simulink model "DTNS_KAISIM_V2"  (R2022a)
settings: Solver=FixedStepDiscrete  StartTime=0.0  StopTime=500  FixedStep=0.04  RelTol=1e-3
PreLoadFcn:
  | listing = dir;
  | if (contains([listing .name], 'DTNS_KAISIM_V2.slx'))
  |     addpath('./TCAF', './TRN', './FTG', './DYN', './FLCC', './GPS', './RALT', './INS', './MAP', './AGR');
  | else
  | 
  | end
  | 
  | load('BUS_STRUCTURE_DYN.mat');
  | load('BUS_STRUCTURE_FLCC.mat');
  | load('BUS_STRUCTURE_RALT.mat');
  | load('BUS_STRUCTURE_INS.mat');
  | load('BUS_STRUCTURE_GPS.mat');
  | load('BUS_STRUCTURE_SENSOR_INPUT.mat');
  | load('BusStructureTRN.mat');
  | load('BusStructureWTPG.mat');
  | load('BusStructureDTF.mat');
  | load('BusStructureGCAWS.mat');
  | load('BusStructureCR.mat');
  | load('BusStructureHR.mat');
  | load('BusStructureLOSR.mat');
  | 
  | clear logsout
InitFcn:
  | listing = dir;
  | if (contains([listing .name], 'DTNS_KAISIM_V2.slx'))
  |     addpath('./TCAF', './TRN', './FTG', './DYN', './FLCC', './GPS', './RALT', './INS', './MAP', './AGR');
  | else
  | 
  | end
  | 
  | load('BUS_STRUCTURE_DYN.mat');
  | load('BUS_STRUCTURE_FLCC.mat');
  | load('BUS_STRUCTURE_RALT.mat');
  | load('BUS_STRUCTURE_INS.mat');
  | load('BUS_STRUCTURE_GPS.mat');
  | load('BUS_STRUCTURE_SENSOR_INPUT.mat');
  | load('BusStructureTRN.mat');
  | load('BusStructureWTPG.mat');
  | load('BusStructureDTF.mat');
  | load('BusStructureGCAWS.mat');
  | load('BusStructureCR.mat');
  | load('BusStructureHR.mat');
  | load('BusStructureLOSR.mat');
  | 
  | clear logsout
(part 2 of 2)

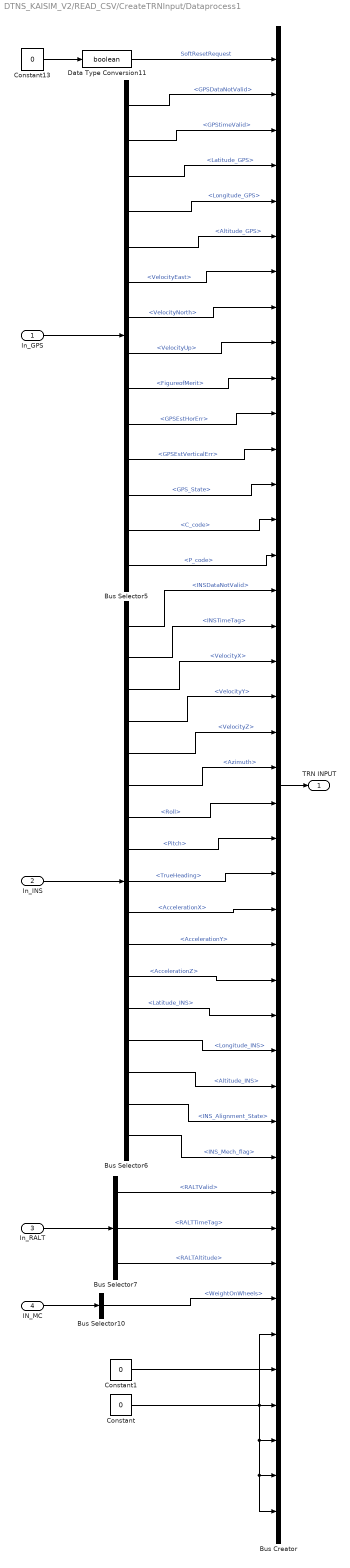
== system DTNS_KAISIM_V2/READ_CSV/CreateTRNInput/Dataprocess1 ==
  In_GPS : Inport
  In_INS : Inport  Port=2
  In_RALT : Inport  Port=3
  IN_MC : Inport  Port=4
  Bus Creator : BusCreator  Inputs=42  OutDataTypeStr=Bus: TRNInput
      settings: InheritFromInputs=off
  Bus Selector10 : BusSelector  OutputSignals=WeightOnWheels
  Bus Selector5 : BusSelector  OutputSignals=GPSDataNotValid,GPStimeValid,Latitude_GPS,Longitude_GPS,Altitude_GPS,VelocityEast,VelocityNorth,VelocityUp,FigureofMerit,GPSEstHorErr,GPSEstVerticalErr,GPS_State,C_code,P_code
  Bus Selector6 : BusSelector  OutputSignals=INSDataNotValid,INSTimeTag,VelocityX,VelocityY,VelocityZ,Azimuth,Roll,Pitch,TrueHeading,AccelerationX,AccelerationY,AccelerationZ,Latitude_INS,Longitude_INS,Altitude_INS,INS_Alignment_State,INS_Mech_flag
  Bus Selector7 : BusSelector  OutputSignals=RALTValid,RALTTimeTag,RALTAltitude
  Constant : Constant  Value=0
  Constant1 : Constant  Value=0  OutDataTypeStr=uint32
  Constant13 : Constant  Value=0
  Data Type Conversion11 : DataTypeConversion  OutDataTypeStr=boolean  SaturateOnIntegerOverflow=off  RndMeth=Floor
  TRN INPUT : Outport  OutDataTypeStr=Bus: TRNInput  VectorParamsAs1DForOutWhenUnconnected=off
  wires:
  Bus Selector6/4 -> Bus Creator/19  "<VelocityY>"
  Bus Selector6/5 -> Bus Creator/20  "<VelocityZ>"
  Bus Selector6/7 -> Bus Creator/22  "<Roll>"
  Bus Selector6/6 -> Bus Creator/21  "<Azimuth>"
  Bus Creator/1 -> TRN INPUT/1
  Bus Selector7/2 -> Bus Creator/34  "<RALTTimeTag>"
  Bus Selector7/1 -> Bus Creator/33  "<RALTValid>"
  Bus Selector6/16 -> Bus Creator/31  "<INS_Alignment_State>"
  Bus Selector5/2 -> Bus Creator/3  "<GPStimeValid>"
  Bus Selector5/1 -> Bus Creator/2  "<GPSDataNotValid>"
  Bus Selector10/1 -> Bus Creator/36  "<WeightOnWheels>"
  Constant/1 -> Bus Creator/41, Bus Creator/42, Bus Creator/40, Bus Creator/37, Bus Creator/39
  Constant13/1 -> Data Type Conversion11/1
  Constant1/1 -> Bus Creator/38
  Bus Selector7/3 -> Bus Creator/35  "<RALTAltitude>"
  Bus Selector6/17 -> Bus Creator/32  "<INS_Mech_flag>"
  Bus Selector6/12 -> Bus Creator/27  "<AccelerationZ>"
  Bus Selector6/13 -> Bus Creator/28  "<Latitude_INS>"
  Bus Selector6/14 -> Bus Creator/29  "<Longitude_INS>"
  Bus Selector6/15 -> Bus Creator/30  "<Altitude_INS>"
  Bus Selector6/8 -> Bus Creator/23  "<Pitch>"
  Bus Selector6/9 -> Bus Creator/24  "<TrueHeading>"
  Bus Selector6/10 -> Bus Creator/25  "<AccelerationX>"
  Bus Selector6/11 -> Bus Creator/26  "<AccelerationY>"
  Bus Selector5/5 -> Bus Creator/6  "<Altitude_GPS>"
  Bus Selector5/6 -> Bus Creator/7  "<VelocityEast>"
  Bus Selector5/4 -> Bus Creator/5  "<Longitude_GPS>"
  Bus Selector5/3 -> Bus Creator/4  "<Latitude_GPS>"
  Bus Selector6/1 -> Bus Creator/16  "<INSDataNotValid>"
  Bus Selector6/2 -> Bus Creator/17  "<INSTimeTag>"
  Bus Selector6/3 -> Bus Creator/18  "<VelocityX>"
  Bus Selector5/11 -> Bus Creator/12  "<GPSEstVerticalErr>"
  Bus Selector5/12 -> Bus Creator/13  "<GPS_State>"
  Bus Selector5/13 -> Bus Creator/14  "<C_code>"
  Bus Selector5/14 -> Bus Creator/15  "<P_code>"
  Bus Selector5/7 -> Bus Creator/8  "<VelocityNorth>"
  Bus Selector5/8 -> Bus Creator/9  "<VelocityUp>"
  Bus Selector5/9 -> Bus Creator/10  "<FigureofMerit>"
  Bus Selector5/10 -> Bus Creator/11  "<GPSEstHorErr>"
  IN_MC/1 -> Bus Selector10/1
  In_RALT/1 -> Bus Selector7/1
  In_INS/1 -> Bus Selector6/1
  In_GPS/1 -> Bus Selector5/1
  Data Type Conversion11/1 -> Bus Creator/1  "SoftResetRequest"

== matlab function DTNS_KAISIM_V2/READ_CSV/CreateTRNSensorMCInput/getPLTF2Body ==
  data: vec_p input; C_pb output; alpha input; rpy input; vec_b output
function [C_pb, vec_b] = getPLTF2Body(vec_p, alpha, rpy)
%getPLTF2Body Convert a vector in INS Platform axis to body frame
%
% Inputs
%   vec_p   : a vector in INS platform axis (3x1)
%   alpha   : wander angle "platform azimuth - true heading" (deg)
%   rpy     : roll, pitch, yaw(true heading) angles (deg)
%
% Outputs
%   C_pb    : computed tranformation matrix from INS Platform axis to body 
% axis
%   vec_b   : converted vec_p in in body frame

% Initialize
C_pb = zeros(3,3);
vec_b = zeros(3,1);

% Arrange
cRol = cosd(rpy(1));
sRol = sind(rpy(1));
cPit = cosd(rpy(2));
sPit = sind(rpy(2));
cYaw = cosd(rpy(3));
sYaw = sind(rpy(3));

% Transformation matrix from INS Platform axis to local NED navigation
% frame
C_pn = [ cosd(alpha), -sind(alpha),  0; ...
        -sind(alpha), -cosd(alpha),  0; ...
                   0,            0, -1];

% Transformation matrix from local NED to body
C_nb = [               cPit*cYaw,                cPit*sYaw,     -sPit;...
        sRol*sPit*cYaw-cRol*sYaw, sRol*sPit*sYaw+cRol*cYaw, sRol*cPit;...
        cRol*sPit*cYaw+sRol*sYaw, cRol*sPit*sYaw-sRol*cYaw, cRol*cPit];


% Convert a given vector to body
vec_b = C_nb * C_pn * vec_p;

end

== matlab function DTNS_KAISIM_V2/InitNUpdateMapCache/UpdateCache/UpdateCache ==
  data: result output; INS_Latitude_Deg input; INS_Longitude_Deg input; TRN_Latitude_Deg input; TRN_Longitude_Deg input
function result = UpdateCache(INS_Latitude_Deg, INS_Longitude_Deg, TRN_Latitude_Deg, TRN_Longitude_Deg)
%UpdateCache

% Persistent variables
persistent firstRun latPrev lonPrev
if isempty(firstRun)
    firstRun = true;
end
if isempty(latPrev)
    latPrev = 0.0;
end
if isempty(lonPrev)
    lonPrev = 0.0;
end

% Initialize output
result = int32(1);
if (firstRun)
    result = coder.ceval('UpdateCache', INS_Latitude_Deg, INS_Longitude_Deg);
    latPrev = INS_Latitude_Deg;
    lonPrev = INS_Longitude_Deg;
    firstRun = false;
elseif (~firstRun) && ( ( abs(TRN_Latitude_Deg - latPrev) > 0.05 ) || ( abs(TRN_Longitude_Deg - lonPrev) > 0.05) )
    result = coder.ceval('UpdateCache', TRN_Latitude_Deg, TRN_Longitude_Deg);
    latPrev = TRN_Latitude_Deg;
    lonPrev = TRN_Longitude_Deg;
else
    
end

== matlab function DTNS_KAISIM_V2/LogData_process/InitUpdateMapCache/Caching/FTGMapCaching1 ==
  data: resultDTED output; resultDVOF output; lat input; lon input; hDEM output
function [resultDTED, resultDVOF, hDEM] = FTGMapCaching(lat, lon)

resultDTED = uint32(1);
resultDVOF = int32(1);
hDEM = double(0.0);                                 %%20220419

resultDTED = coder.ceval('UpdateMapCache', lat, lon);
hDEM = coder.ceval('MAPGetTerrainHeight', lat, lon);       %%20220419

== matlab function DTNS_KAISIM_V2/InitNUpdateMapCache/InitializeMAP ==
  data: successDTED output; successDVOF output
function [successDTED, successDVOF] = InitializeMAP()
%InitializeMAP

% Persistent variable
persistent firstRun
if isempty(firstRun)
    firstRun = true;
end

% Initialize output
flagDTED = int32(1);
flagDVOF = int32(1);
successDTED = int32(1);
successDVOF = int32(1);

if firstRun
    % Path of DTED data
    pathDTED = 'C:\Users\ASCL\Documents\GitHub\DTNS\MAP\MAP_DB';

    % Length of DETD data path
    strLenDTED = int32(strlength(pathDTED));
    
    % Call [ InitialMap ] : 맵 폴더 위치 설정
    flagDTED = coder.ceval('InitialMap', pathDTED, strLenDTED );
    
    successDTED = flagDTED;

    if (successDTED)
        firstRun = false;
    end
else
    successDTED = int32(0);
    successDVOF = int32(0);
end

== matlab function DTNS_KAISIM_V2/MATFunction_VisualizeWCP ==
  data: wtp input; predictedTraj input; pathDTF input; pathGCAWS input
function Visualize(wtp, predictedTraj, pathDTF, pathGCAWS)
%VISUALIZE
% 
persistent fHandle subPlot1 subPlot2 tSpanWCP tSpanPT count map ARCSEC2DEG mapSurf predBound yAxisMax

acXY = zeros(2,27);
heading = 0;

% Initialize Figure Handle
if isempty(fHandle)
    fHandle = figure('WindowStyle', 'docked');
end

% Divide and Initailize the Figure
if isempty(subPlot1)
    set(0, 'CurrentFigure', fHandle);
    subPlot1 = subplot(1, 4, 1:2);
    axis equal;
    colormap(fliplr(hsv));
    view(0, 90);
    set(gca, 'Color', [0.3, 0.3, 0.3]);
    xlabel('Longitude [deg]');
    ylabel('Latitude [deg]');
    hold off;
end

% Divide and Initailize the Figure
if isempty(subPlot2)
    subPlot2 = subplot(1, 4, 3:4);
    hold on;
    grid minor;
    xlabel('Time [sec]');
    ylabel('Height [m]');
    axis([-0.5, 20, 0, 2000]);
    hold off;
end

% Initialize tSpanWCP
if isempty(tSpanWCP)
    tSpanWCP = 0:0.5:((length(wtp)-1)*0.5);
end

% Initialize tSpanPT
if isempty(tSpanPT)
    tSpanPT = 0:0.25:((size(predictedTraj, 1)-1)*0.25);
end

% Initialize count
if isempty(count)
    count = 0;    
end

% Initialize yAxisMax
if isempty(yAxisMax) 
    yAxisMax = 2000;
end
% Initialize ARCSEC2DEG
if isempty(ARCSEC2DEG)
    ARCSEC2DEG = (0.000277777777777777);
end

% Initialize map
if isempty(map)
    map = ones(150, 150, 3);

    % Current A/C Position
    latTrue = predictedTraj(1, 1, 1);
    lonTrue = predictedTraj(1, 1, 2);
    
    % Flooring to neighboring Map Grid
    latTrun = floor(latTrue/(3*ARCSEC2DEG)) * (3*ARCSEC2DEG);
    lonTrun = floor(lonTrue/(3*ARCSEC2DEG)) * (3*ARCSEC2DEG);
    
    mapSizeLat = size(map, 1);
    mapSizeLon = size(map, 2);
    % Update map data
    for ii = 1:size(map, 1)
    
        for jj = 1:size(map, 2)
            
            map(ii, jj, 1) = latTrun + (9*ARCSEC2DEG) * ((size(map, 1) - floor(mapSizeLat * 1.5)) + ii);
            map(ii, jj, 2) = lonTrun + (9*ARCSEC2DEG) * ((size(map, 2) - floor(mapSizeLon * 1.5)) + jj);
            
            map(ii, jj, 3) = ...
            coder.ceval('MAPGetTerrainHeight', map(ii, jj, 1), map(ii, jj, 2)); 

            if (ii == size(map, 1)) && (jj == size(map, 2))
                map(ii, jj, 3) = 2200;
            end
            
        end
    
    end
    
end

% Initialize mapSurf: mapSurf plot handle
if isempty(mapSurf)
    set(0, 'CurrentFigure', fHandle);
    subplot(subPlot1);
    hold on;
    mapSurf = surf(map(:,:,2), map(:,:,1), map(:,:,3), 'FaceAlpha', 0.75);
    drawnow;
    hold off;
end

% Initialize predBound: predBound plot handle
if isempty(predBound)
    set(0, 'CurrentFigure', fHandle);
    subplot(subPlot1);
    hold on;
    predBound = plot3([predictedTraj(:,2,2); flipud(predictedTraj(:,3,2))], ...
        [predictedTraj(:,2,1); flipud(predictedTraj(:,3,1))], ...
        [predictedTraj(:,2,3); flipud(predictedTraj(:,3,3))], '-m', 'LineWidth', 3);
    hold off;
end


%%

% Limit & Reset count
if (count >= 250)
    count = 0;
end

% 0.5Hz Event
if rem(count, 50) == 0
    set(0, 'CurrentFigure', fHandle);
    subplot(subPlot1);
    hold on;
    
    % Current A/C Position
    latTrue = predictedTraj(1, 1, 1);
    lonTrue = predictedTraj(1, 1, 2);
    
    % Flooring to neighboring Map Grid
    latTrun = floor(latTrue/(3*ARCSEC2DEG)) * (3*ARCSEC2DEG);
    lonTrun = floor(lonTrue/(3*ARCSEC2DEG)) * (3*ARCSEC2DEG);
    
    mapSizeLat = size(map, 1);
    mapSizeLon = size(map, 2);
    if abs(latTrun-(map(1, 1, 1)+map(end, 1, 1))/2) >= 100*(3*ARCSEC2DEG) || abs(lonTrun-(map(1, 1, 2)+map(1, end, 2))/2) >= 100*(3*ARCSEC2DEG)
        % Update map data
        for ii = 1:size(map, 1)
            for jj = 1:size(map, 2)
                map(ii, jj, 1) = latTrun + (9*ARCSEC2DEG) * ((size(map, 1) - floor(mapSizeLat * 1.5)) + ii);
                map(ii, jj, 2) = lonTrun + (9*ARCSEC2DEG) * ((size(map, 2) - floor(mapSizeLon * 1.5)) + jj);
                map(ii, jj, 3) = ...
                coder.ceval('MAPGetTerrainHeight', map(ii, jj, 1), map(ii, jj, 2)); 
            end
        end
        
        set(mapSurf, 'XData', map(:,:,2), 'YData', map(:,:,1), 'ZData', map(:,:,3));
        drawnow;
    end
    
    % Draw Map
    axis([lonTrun - (3*ARCSEC2DEG)*60, lonTrun + (3*ARCSEC2DEG)*60, latTrun - (3*ARCSEC2DEG)*60, latTrun + (3*ARCSEC2DEG)*60]);
    drawnow;
    hold off;
    
end

% 2.5Hz Event
if rem(count, 5) == 0
    set(0, 'CurrentFigure', fHandle);
    subplot(subPlot1);
    
    hold on;
    latTrue = predictedTraj(1, 1, 1);
    lonTrue = predictedTraj(1, 1, 2);
    heading = getHeadingFromVector([latTrue, lonTrue], [predictedTraj(81, 1, 1), predictedTraj(81, 1, 2)]);
    acXY = drawAircraft( [lonTrue;latTrue], 4.5*ARCSEC2DEG, heading);
    plot3(acXY(1,:), acXY(2,:), predictedTraj(1, 1, 3)*ones(size(acXY(1,:))), '-r')
    
    set(predBound, 'XData', [predictedTraj(:,2,2); flipud(predictedTraj(:,3,2))], ...
    'YData', [predictedTraj(:,2,1); flipud(predictedTraj(:,3,1))], ...
    'ZData', [predictedTraj(:,2,3); flipud(predictedTraj(:,3,3))]);
    
    hold off;
    
    set(0, 'CurrentFigure', fHandle);
    subplot(subPlot2);
    
    nominalTerrain = zeros(size(predictedTraj, 1), 1);
    for nn = 1:size(predictedTraj(:,1,3), 1)
        nominalTerrain(nn) = coder.ceval('MAPGetTerrainHeight', predictedTraj(nn, 1, 1), predictedTraj(nn, 1, 2)); 
    end
    
    hold on;
    cla
    plot(tSpanPT, nominalTerrain, '-g', 'LineWidth', 5, 'DisplayName', 'Nominal Terrain');
    plot(tSpanWCP, wtp, '-b', 'LineWidth', 5, 'DisplayName', 'WCP');
    plot(tSpanPT, predictedTraj(:, 1, 3), '--k', 'LineWidth', 2, 'DisplayName', 'Predicted Nominal Trajectory');
    plot(0, predictedTraj(1, 1, 3), 'ro', 'MarkerSize', 10, 'DisplayName', 'A/C');
    plot(0:0.5:20, pathDTF, '-y', 'DisplayName','DBTF Reference Trajectory', 'LineWidth', 2);
    
    for ii = 1:12
       plot(0:0.5:20, pathGCAWS(:,ii,3));
       
    end
    
    if (predictedTraj(1, 1, 3) > yAxisMax-300)
        axis([-0.5, 20, 0, predictedTraj(1, 1, 3) + 500]);
    elseif (predictedTraj(1, 1, 3) < 1800)
        axis([-0.5, 20, 0, 2000])
    end
    % axis([-1, 20, 300, 800]);
    drawnow;
    hold off; 
    
end

% Update count
count = count + 1;

end


function [acXY] = drawAircraft(centerXY, longLength, heading)
%DRAWAircraft
    % centerXY      (2x1)
    % longLength    (1) [deg]
    % heading       (1) [deg]
    
    acXY = zeros(2, 27);
    translate = ones(2, 27);
    translate(1,:) = translate(1,:) * centerXY(1); 
    translate(2,:) = translate(2,:) * centerXY(2); 
    
    refXY = [ 0, -2, -4, -6,-16,-16,-17,-17, -4, -4, -9,-10, -4,  0,  4, 10,  9,  4,  4, 17, 17, 16, 16,  6,  4,  2,  0;...
             25, 20,  8,  0, -7, -4, -4,-14,-14,-18,-23,-26,-25,-25,-25,-26,-23,-18,-14,-14, -4, -4, -7,  0,  8, 20, 25];
    
    acXY = refXY / 50 * longLength;
    
    rot = [cosd(-heading), -sind(-heading); sind(-heading), cosd(-heading)];
    
    acXY = rot * acXY + translate;
    
end

function [heading] = getHeadingFromVector(fromLatLon, toLatLon)
%GETHEADINGFROMVECTOR
    % fromLatLon (2x1) [deg]
    % toLatLon (2x1) [deg]
    
    dLon = toLatLon(2) - fromLatLon(2);
    
    y = sind(dLon) * cosd(toLatLon(1));
    x = cosd(fromLatLon(1)) * sind(toLatLon(1)) ...
        - sind(fromLatLon(1)) * cosd(toLatLon(1)) * cosd(dLon);
    
    heading = atan2d(y, x);
    heading = rem( heading + 360, 360);

end

== matlab function DTNS_KAISIM_V2/READ_CSV/Subsystem2/getPLTF2Body ==
  data: vec_p input; C_pb output; alpha input; rpy input; vec_b output
function [C_pb, vec_b] = getPLTF2Body(vec_p, alpha, rpy)
%getPLTF2Body Convert a vector in INS Platform axis to body frame
%
% Inputs
%   vec_p   : a vector in INS platform axis (3x1)
%   alpha   : wander angle "platform azimuth - true heading" (deg)
%   rpy     : roll, pitch, yaw(true heading) angles (deg)
%
% Outputs
%   C_pb    : computed tranformation matrix from INS Platform axis to body 
% axis
%   vec_b   : converted vec_p in in body frame

% Initialize
C_pb = zeros(3,3);
vec_b = zeros(3,1);

% Arrange
cRol = cosd(rpy(1));
sRol = sind(rpy(1));
cPit = cosd(rpy(2));
sPit = sind(rpy(2));
cYaw = cosd(rpy(3));
sYaw = sind(rpy(3));

% Transformation matrix from INS Platform axis to local NED navigation
% frame
C_pn = [ cosd(alpha), -sind(alpha),  0; ...
        -sind(alpha), -cosd(alpha),  0; ...
                   0,            0, -1];

% Transformation matrix from local NED to body
C_nb = [               cPit*cYaw,                cPit*sYaw,     -sPit;...
        sRol*sPit*cYaw-cRol*sYaw, sRol*sPit*sYaw+cRol*cYaw, sRol*cPit;...
        cRol*sPit*cYaw+sRol*sYaw, cRol*sPit*sYaw-sRol*cYaw, cRol*cPit];


% Convert a given vector to body
vec_b = C_nb * C_pn * vec_p;

end

== matlab function DTNS_KAISIM_V2/VisualizeWTPOnly ==
  data: wtp input; predictedTraj input
function VisualizeWTPOnly(wtp, predictedTraj)
%VisualizeWTPOnly
% 
persistent fHandle subPlot1 subPlot2 tSpanWCP tSpanPT count map ARCSEC2DEG mapSurf predBound yAxisMax

acXY = zeros(2,27);
heading = 0;

% Initialize Figure Handle
if isempty(fHandle)
    fHandle = figure('WindowStyle', 'docked');
end

% Divide and Initailize the Figure
if isempty(subPlot1)
    set(0, 'CurrentFigure', fHandle);
%     subPlot1 = subplot(5, 1, 1:4, 'position', [0.05 0.525 0.9 0.425]);
    subPlot1 = subplot(1, 4, 1:2);
    axis equal;
    colormap(fliplr(hsv));
    view(0, 90);
    set(gca, 'Color', [0.3, 0.3, 0.3]);
    xlabel('Longitude [deg]');
    ylabel('Latitude [deg]');
    hold off;
end

% Divide and Initailize the Figure
if isempty(subPlot2)
%     subPlot2 = subplot(5, 1, 5, 'position', [0.1 0.05 0.8 0.425]);
    subPlot2 = subplot(1, 4, 3:4);
    hold on;
    grid minor;
    xlabel('Time [sec]');
    ylabel('Height [m]');
    axis([-0.5, 20, 0, 2000]);
    hold off;
end

% Initialize tSpanWCP
if isempty(tSpanWCP)
    tSpanWCP = 0:0.5:((length(wtp)-1)*0.5);
end

% Initialize tSpanPT
if isempty(tSpanPT)
    tSpanPT = 0:0.25:((size(predictedTraj, 1)-1)*0.25);
end

% Initialize count
if isempty(count)
    count = 0;    
end

% Initialize yAxisMax
if isempty(yAxisMax) 
    yAxisMax = 2000;
end
% Initialize ARCSEC2DEG
if isempty(ARCSEC2DEG)
    ARCSEC2DEG = (0.000277777777777777);
end

% Initialize map
if isempty(map)
    map = ones(150, 150, 3);

    % Current A/C Position
    latTrue = predictedTraj(1, 1, 1);
    lonTrue = predictedTraj(1, 1, 2);
    
    % Flooring to neighboring Map Grid
    latTrun = floor(latTrue/(3*ARCSEC2DEG)) * (3*ARCSEC2DEG);
    lonTrun = floor(lonTrue/(3*ARCSEC2DEG)) * (3*ARCSEC2DEG);
    
    mapSizeLat = size(map, 1);
    mapSizeLon = size(map, 2);
    % Update map data
    for ii = 1:size(map, 1)
    
        for jj = 1:size(map, 2)
            
            map(ii, jj, 1) = latTrun + (9*ARCSEC2DEG) * ((size(map, 1) - floor(mapSizeLat * 1.5)) + ii);
            map(ii, jj, 2) = lonTrun + (9*ARCSEC2DEG) * ((size(map, 2) - floor(mapSizeLon * 1.5)) + jj);
            
            map(ii, jj, 3) = ...
            coder.ceval('MAPGetTerrainHeight', map(ii, jj, 1), map(ii, jj, 2)); 
            if (ii == size(map, 1)) && (jj == size(map,2))
                map(ii, jj, 3) = 2000;
            end
            
        end
    
    end
    
end

% Initialize mapSurf: mapSurf plot handle
if isempty(mapSurf)
    set(0, 'CurrentFigure', fHandle);
    subplot(subPlot1);
    hold on;
    mapSurf = surf(map(:,:,2), map(:,:,1), map(:,:,3), 'FaceAlpha', 0.85);
    drawnow;
    hold off;
end

% Initialize predBound: predBound plot handle
if isempty(predBound)
    set(0, 'CurrentFigure', fHandle);
    subplot(subPlot1);
    hold on;
    predBound = plot3([predictedTraj(:,2,2); flipud(predictedTraj(:,3,2))], ...
        [predictedTraj(:,2,1); flipud(predictedTraj(:,3,1))], ...
        [predictedTraj(:,2,3); flipud(predictedTraj(:,3,3))], '-m', 'LineWidth', 3);
    hold off;
end


%%

% Limit & Reset count
if (count >= 250)
    count = 0;
end

% 5Hz Event
if rem(count, 5) == 0
    set(0, 'CurrentFigure', fHandle);
    subplot(subPlot1);
    hold on;
    
    % Current A/C Position
    latTrue = predictedTraj(1, 1, 1);
    lonTrue = predictedTraj(1, 1, 2);
    
    % Flooring to neighboring Map Grid
    latTrun = floor(latTrue/(3*ARCSEC2DEG)) * (3*ARCSEC2DEG);
    lonTrun = floor(lonTrue/(3*ARCSEC2DEG)) * (3*ARCSEC2DEG);
    
    mapSizeLat = size(map, 1);
    mapSizeLon = size(map, 2);
    if abs(latTrun-(map(1, 1, 1)+map(end, 1, 1))/2) >= 100*(3*ARCSEC2DEG) || abs(lonTrun-(map(1, 1, 2)+map(1, end, 2))/2) >= 100*(3*ARCSEC2DEG)
        % Update map data
        for ii = 1:size(map, 1)
            for jj = 1:size(map, 2)
                map(ii, jj, 1) = latTrun + (9*ARCSEC2DEG) * ((size(map, 1) - floor(mapSizeLat * 1.5)) + ii);
                map(ii, jj, 2) = lonTrun + (9*ARCSEC2DEG) * ((size(map, 2) - floor(mapSizeLon * 1.5)) + jj);
                map(ii, jj, 3) = ...
                coder.ceval('MAPGetTerrainHeight', map(ii, jj, 1), map(ii, jj, 2)); 
            end
        end
        
        set(mapSurf, 'XData', map(:,:,2), 'YData', map(:,:,1), 'ZData', map(:,:,3));
        drawnow;
    end
    
    % Draw Map
    axis([lonTrun - (3*ARCSEC2DEG)*60, lonTrun + (3*ARCSEC2DEG)*60, latTrun - (3*ARCSEC2DEG)*60, latTrun + (3*ARCSEC2DEG)*60]);
    drawnow;
    hold off;
    
end

% 2.5Hz Event
if rem(count, 5) == 0
    set(0, 'CurrentFigure', fHandle);
    subplot(subPlot1);
    
    hold on;
    latTrue = predictedTraj(1, 1, 1);
    lonTrue = predictedTraj(1, 1, 2);
    heading = getHeadingFromVector([latTrue, lonTrue], [predictedTraj(81, 1, 1), predictedTraj(81, 1, 2)]);
    acXY = drawAircraft( [lonTrue;latTrue], 4.5*ARCSEC2DEG, heading);
    plot3(acXY(1,:), acXY(2,:), predictedTraj(1, 1, 3)*ones(size(acXY(1,:))), '-r')
    
    set(predBound, 'XData', [predictedTraj(:,2,2); flipud(predictedTraj(:,3,2))], ...
    'YData', [predictedTraj(:,2,1); flipud(predictedTraj(:,3,1))], ...
    'ZData', [predictedTraj(:,2,3); flipud(predictedTraj(:,3,3))]+200);
    
    hold off;
    
    set(0, 'CurrentFigure', fHandle);
    subplot(subPlot2);
    
    nominalTerrain = zeros(size(predictedTraj, 1), 1);
    for nn = 1:size(predictedTraj(:,1,3), 1)
        nominalTerrain(nn) = coder.ceval('MAPGetTerrainHeight', predictedTraj(nn, 1, 1), predictedTraj(nn, 1, 2)); 
    end
    
    hold on;
    cla
    plot(tSpanPT, nominalTerrain, '-g', 'LineWidth', 5, 'DisplayName', 'Nominal Terrain');
    plot(tSpanWCP, wtp, '-b', 'LineWidth', 5, 'DisplayName', 'WCP');

    if (predictedTraj(1, 1, 3) > yAxisMax-300)
        axis([-0.5, 20, 0, predictedTraj(1, 1, 3) + 500]);
    elseif (predictedTraj(1, 1, 3) < 1800)
        axis([-0.5, 20, 0, 2000])
    end
    % axis([-1, 20, 300, 800]);
    drawnow;
    hold off; 
    
end

% Update count
count = count + 1;

end


function [acXY] = drawAircraft(centerXY, longLength, heading)
%DRAWAircraft
    % centerXY      (2x1)
    % longLength    (1) [deg]
    % heading       (1) [deg]
    
    acXY = zeros(2, 27);
    translate = ones(2, 27);
    translate(1,:) = translate(1,:) * centerXY(1); 
    translate(2,:) = translate(2,:) * centerXY(2); 
    
    refXY = [ 0, -2, -4, -6,-16,-16,-17,-17, -4, -4, -9,-10, -4,  0,  4, 10,  9,  4,  4, 17, 17, 16, 16,  6,  4,  2,  0;...
             25, 20,  8,  0, -7, -4, -4,-14,-14,-18,-23,-26,-25,-25,-25,-26,-23,-18,-14,-14, -4, -4, -7,  0,  8, 20, 25];
    
    acXY = refXY / 50 * longLength;
    
    rot = [cosd(-heading), -sind(-heading); sind(-heading), cosd(-heading)];
    
    acXY = rot * acXY + translate;
    
end

function [heading] = getHeadingFromVector(fromLatLon, toLatLon)
%GETHEADINGFROMVECTOR
    % fromLatLon (2x1) [deg]
    % toLatLon (2x1) [deg]
    
    dLon = toLatLon(2) - fromLatLon(2);
    
    y = sind(dLon) * cosd(toLatLon(1));
    x = cosd(fromLatLon(1)) * sind(toLatLon(1)) ...
        - sind(fromLatLon(1)) * cosd(toLatLon(1)) * cosd(dLon);
    
    heading = atan2d(y, x);
    heading = rem( heading + 360, 360);

end

== matlab function DTNS_KAISIM_V2/LogData_process/InitUpdateMapCache/InitializeMAP ==
  data: successDTED output; successDVOF output
function [successDTED, successDVOF] = InitializeMAP()
%InitializeMAP

% Persistent variable
persistent firstRun
if isempty(firstRun)
    firstRun = true;
end

% Initialize output
flagDTED = int32(1);
flagDVOF = int32(1);
successDTED = int32(1);
successDVOF = int32(1);

if firstRun
    % Path of DTED data
    pathDTED = 'C:\MAP2\MAP_DB\';

    % Length of DETD data path
    strLenDTED = int32(strlength(pathDTED));
    
    % Call [ InitialMap ] : 맵 폴더 위치 설정
    flagDTED = coder.ceval('InitialMap', pathDTED, strLenDTED );
    
    successDTED = flagDTED;

    if (successDTED)
        firstRun = false;
    end
else
    successDTED = int32(0);
    successDVOF = int32(0);
end

== matlab function DTNS_KAISIM_V2/ConvertBodyToPlatform ==
  data: vecBodyXYZ input; vecPlatformXYZ output; az_rad input
function vecPlatformXYZ = ConvertBodyToPlatform(vecBodyXYZ, az_rad)
%CONVERTBODYTOPLATFORM

vecPlatformXYZ = zeros(3, 1);

tformMat = diag([1, -1, -1]) * ...
    [cos(az_rad), -sin(az_rad), 0; ...
     sin(az_rad), cos(az_rad), 0; ...
     0, 0, 1];

vecPlatformXYZ = tformMat * vecBodyXYZ;

== matlab function DTNS_KAISIM_V2/ConvertPlatformToBody ==
  data: vecPlatformXYZ input; vecBodyXYZ output; az_rad input
function vecBodyXYZ = ConvertPlatformToBody(vecPlatformXYZ, az_rad)
%CONVERTBODYTOPLATFORM

vecBodyXYZ = zeros(3, 1);

tformMat = diag([1, -1, -1]) * ...
    [cos(az_rad), -sin(az_rad), 0; ...
     sin(az_rad), cos(az_rad), 0; ...
     0, 0, 1];

tformMat = tformMat';

vecBodyXYZ = tformMat * vecPlatformXYZ;

== matlab function DTNS_KAISIM_V2/READ_CSV/CreateTRNSensorMCInput/getPLTF2Body1 ==
  data: vec_p input; C_pb output; alpha input; rpy input; vec_b output
function [C_pb, vec_b] = getPLTF2Body(vec_p, alpha, rpy)
%getPLTF2Body Convert a vector in INS Platform axis to body frame
%
% Inputs
%   vec_p   : a vector in INS platform axis (3x1)
%   alpha   : wander angle "platform azimuth - true heading" (deg)
%   rpy     : roll, pitch, yaw(true heading) angles (deg)
%
% Outputs
%   C_pb    : computed tranformation matrix from INS Platform axis to body 
% axis
%   vec_b   : converted vec_p in in body frame

% Initialize
C_pb = zeros(3,3);
vec_b = zeros(3,1);

% Arrange
cRol = cosd(rpy(1));
sRol = sind(rpy(1));
cPit = cosd(rpy(2));
sPit = sind(rpy(2));
cYaw = cosd(rpy(3));
sYaw = sind(rpy(3));

% Transformation matrix from INS Platform axis to local NED navigation
% frame
C_pn = [ cosd(alpha), -sind(alpha),  0; ...
        -sind(alpha), -cosd(alpha),  0; ...
                   0,            0, -1];

% Transformation matrix from local NED to body
C_nb = [               cPit*cYaw,                cPit*sYaw,     -sPit;...
        sRol*sPit*cYaw-cRol*sYaw, sRol*sPit*sYaw+cRol*cYaw, sRol*cPit;...
        cRol*sPit*cYaw+sRol*sYaw, cRol*sPit*sYaw-sRol*cYaw, cRol*cPit];


% Convert a given vector to body
vec_b = C_nb * C_pn * vec_p;

end

== matlab function DTNS_KAISIM_V2/AGR/BallisticComputer ==
  data: TRNOutput input Bus: TRNOutput; IN_HRInput input; selected output; HRDataTag output; rangeN output; rangeE output; targetElev input; Valid input
function [selected, HRDataTag, rangeN, rangeE] = BallisticComputer(TRNOutput, IN_HRInput, targetElev, Valid)
%BallisticComputer

% Initialize outputs
selected = true;
rangeN = 0.0;
rangeE = 0.0;

x = 0.0;
z = 0.0;

HRDataTag = IN_HRInput.HRDataTag;

% Rearrange variables
llh = [TRNOutput.TRNEstOfLatitude; ...
    TRNOutput.TRNEstOfLongitude; ...
    TRNOutput.Altitude_INS - TRNOutput.TRNEstOfINSAltitudeErr];

velXYZ = [TRNOutput.TRN_VelocityX; ...
    TRNOutput.TRN_VelocityY; ...
    TRNOutput.TRN_VelocityZ];

attiDeg = [TRNOutput.TRN_Roll; TRNOutput.TRN_Pitch; TRNOutput.TRN_Yaw];

if Valid
    velNED = body2ned(velXYZ, attiDeg);
    V0 = norm(velNED);
    gamma = atan2d(-velNED(3), sqrt(velNED(1)^2+velNED(2)^2));
    z0 = llh(3);
    x0 = 0;
    T = findTime(double(targetElev), z0, V0, gamma);
    if T >= 0

        heading = atan2d(velNED(2), velNED(1));
        [x, z] = bombKinematics(x0, z0, V0, gamma, T);
        selected = true;
        rangeN = x * cosd(heading);
        rangeE = x * sind(heading);
    else
        selected = false;
        rangeN = 0.0;
        rangeE = 0.0;
    end


else
    selected = true;
    rangeN = 0.0;
    rangeE = 0.0;
end

end

%% Internal functions
function [x, z] = bombKinematics(x0, z0, V0, gamma, t)
    
    g = 9.8;
    x = x0 + V0 * cosd(gamma) .* t;
    z = z0 + V0 * sind(gamma) .* t - 0.5 * g * t.^2;
end

function T = findTime(z, z0, V0, gamma)

g = 9.8;

temp = V0^2*(sind(gamma))^2 - 2*g*(z-z0);

if temp < 0
    T = 0;
else
    T = (V0*sind(gamma) + sqrt(V0^2*(sind(gamma))^2 - 2*g*(z-z0) ) ) / g;
end
end

function [state_eb_n, C_b_n] = body2ned(state_eb_b, eulerDeg)
%body2ned
% Compute the transformation from {Body} frame to local {NED} frame
%
% == Inputs =========
% state_eb_b        - states measured w.r.t. {ECEF} and resolved in {Body}
% eulerDeg          - attitude (euler angles roll-pitch-yaw seq.) [deg]
%
% == Outputs ========
% state_eb_n        - xyz-states resolved in {NED}
% C_b_n             - Transformation matirx from {Body} to {NED} (3x3)
% 

state_eb_n  = zeros(3,1);
C_b_n       = zeros(3,3);

% Body to NED
cRol = cosd(eulerDeg(1));
sRol = sind(eulerDeg(1));
cPit = cosd(eulerDeg(2));
sPit = sind(eulerDeg(2));
cYaw = cosd(eulerDeg(3));
sYaw = sind(eulerDeg(3));
% 
% C_n_b   = [              cPit*cYaw,                cPit*sYaw,     -sPit;...
%           sRol*sPit*cYaw-cRol*sYaw, sRol*sPit*sYaw+cRol*cYaw, sRol*cPit;...
%           cRol*sPit*cYaw+sRol*sYaw, cRol*sPit*sYaw-sRol*cYaw, cRol*cPit];

C_b_n   = [ cPit*cYaw, sRol*sPit*cYaw-cRol*sYaw, cRol*sPit*cYaw+sRol*sYaw;...
            cPit*sYaw, sRol*sPit*sYaw+cRol*cYaw, cRol*sPit*sYaw-sRol*cYaw;...
                -sPit,                sRol*cPit,                cRol*cPit];
% C_b_n   = C_n_b';
      
state_eb_n  = C_b_n * state_eb_b;


end

== matlab function DTNS_KAISIM_V2/READ_CSV/Subsystem2/getPLTF2Body1 ==
  data: vec_p input; C_pb output; alpha input; rpy input; vec_b output
function [C_pb, vec_b] = getPLTF2Body(vec_p, alpha, rpy)
%getPLTF2Body Convert a vector in INS Platform axis to body frame
%
% Inputs
%   vec_p   : a vector in INS platform axis (3x1)
%   alpha   : wander angle "platform azimuth - true heading" (deg)
%   rpy     : roll, pitch, yaw(true heading) angles (deg)
%
% Outputs
%   C_pb    : computed tranformation matrix from INS Platform axis to body 
% axis
%   vec_b   : converted vec_p in in body frame

% Initialize
C_pb = zeros(3,3);
vec_b = zeros(3,1);

% Arrange
cRol = cosd(rpy(1));
sRol = sind(rpy(1));
cPit = cosd(rpy(2));
sPit = sind(rpy(2));
cYaw = cosd(rpy(3));
sYaw = sind(rpy(3));

% Transformation matrix from INS Platform axis to local NED navigation
% frame
C_pn = [ cosd(alpha), -sind(alpha),  0; ...
        -sind(alpha), -cosd(alpha),  0; ...
                   0,            0, -1];

% Transformation matrix from local NED to body
C_nb = [               cPit*cYaw,                cPit*sYaw,     -sPit;...
        sRol*sPit*cYaw-cRol*sYaw, sRol*sPit*sYaw+cRol*cYaw, sRol*cPit;...
        cRol*sPit*cYaw+sRol*sYaw, cRol*sPit*sYaw-sRol*cYaw, cRol*cPit];


% Convert a given vector to body
vec_b = C_nb * C_pn * vec_p;

end
